simulink model "net_model_5_nodes_distributed_controllers"  (R2024b)
settings: Solver=FixedStepAuto  StartTime=0.0  StopTime=n_max  FixedStep=1  RelTol=1e-3
values from neighbouring files (symbols this model uses):
  A_ctrl = zeros(n, n, n_of_systems)    [compute_controller.m]    (also in distributed_sw_stable_ctrl_sparse_slow.mat = [-2.40828892384e-08 -0.401671155219 -3.56889576468e-19 -4.25)
  B_ctrl = -L    [compute_controller.m]    (also in distributed_sw_stable_ctrl_sparse_slow.mat = [1.00000002408 3.28131707351e-09 3.56889576468e-19 -1.412131)
  C_ctrl = J    [compute_controller.m]    (also in distributed_sw_stable_ctrl_sparse_slow.mat = [-0.301574287938 -5.67211227989e-16 -0.0985259199916 4.99277)
  D_ctrl = zeros(m, p, n_of_systems)    [compute_controller.m]    (also in distributed_sw_stable_ctrl_sparse_slow.mat = [0 0 0 0 0 0 0 0 0 0 0 0 ... (450 elements, 5x10x9)])
  n_T_local = 5    [main.m]
  node_1_0 = pi / 180 * [5, 0]'    [main.m]
  node_2_0 = pi / 180 * [-8, 0]'    [main.m]
  node_3_0 = pi / 180 * [2, 0]'    [main.m]
  node_4_0 = pi / 180 * [-8, 0]'    [main.m]
  node_5_0 = pi / 180 * [-3, 0]'    [main.m]
  T_A = zeros(n_states, n_states, n_of_systems)    [compute_controller.m]    (also in distributed_sw_stable_ctrl_sparse_slow.mat = [0 0 0 0 0 0 0 0 0 0 0 0 ... (225 elements, 5x5x9)])
  T_B = zeros(n_states, 10, n_of_systems)    [compute_controller.m]    (also in distributed_sw_stable_ctrl_sparse_slow.mat = [0 0 0 0 0 0 0 0 0 0 0 0 ... (450 elements, 5x10x9)])
  T_C = zeros(5, n_states, n_of_systems)    [compute_controller.m]    (also in distributed_sw_stable_ctrl_sparse_slow.mat = [0 0 0 0 0 0 0 0 0 0 0 0 ... (225 elements, 5x5x9)])
  T_D = zeros(5, 10, n_of_systems)    [compute_controller.m]    (also in distributed_sw_stable_ctrl_sparse_slow.mat = [0 0 0 0 0 0 0 0 0 0 0 0 ... (450 elements, 5x10x9)]; main.m)
undefined symbols (not defined in the file or in its folder): a, A_matrices, B, C
(part 2 of 2)

== matlab function net_model_5_nodes_distributed_controllers/Node 1/Interface ==
  data: delta_2 input; delta_3 input; delta_5 input; neigh_values output; l_1q input
function neigh_values = fcn(delta_2, delta_3, delta_5, l_1q)

    neigh_values = l_1q(2) * delta_2 + l_1q(3) * delta_3 + l_1q(5) * delta_5;

end

== matlab function net_model_5_nodes_distributed_controllers/Node 1/Node dynamics ==
  data: x_prev input; u input; x output; w input; neigh_values input; l_iq input; current_node input
function x = fcn(x_prev, u, w, neigh_values, l_iq, current_node)
    
    % current_node = 1;

%%

    hi = [0.3244
        1.5886;
        0.6224;
        1.0571;
        0.3313];

    di = [0.5650;
        0.7844;
        0.7347;
        0.5060;
        0.6686];

    dt = 0.2;
%%

    a21 = -hi(current_node) * dt * sum(l_iq);
    a22 = 1 - hi(current_node) * di(current_node) * dt;

    A = [1, dt;
        a21, a22];

    x = A * x_prev + [0 1]' * (u + w + hi(current_node) * dt * neigh_values);
    
end

== matlab function net_model_5_nodes_distributed_controllers/Node 3/Interface ==
  data: delta_1 input; neigh_values output; delta_4 input; delta_5 input; l_3q input
function neigh_values = fcn(delta_1, delta_4, delta_5, l_3q)

    neigh_values = l_3q(1) * delta_1 + l_3q(4) * delta_4 + l_3q(5) * delta_5;

end

== matlab function net_model_5_nodes_distributed_controllers/Node 3/Node dynamics ==
  data: x_prev input; u input; x output; w input; neigh_values input; l_iq input; current_node input
function x = fcn(x_prev, u, w, neigh_values, l_iq, current_node)
    
    % current_node = 1;

%%

    hi = [0.3244
        1.5886;
        0.6224;
        1.0571;
        0.3313];

    di = [0.5650;
        0.7844;
        0.7347;
        0.5060;
        0.6686];
    dt = 0.2;
%%

    a21 = -hi(current_node) * dt * sum(l_iq);
    a22 = 1 - hi(current_node) * di(current_node) * dt;

    A = [1, dt;
        a21, a22];

    x = A * x_prev + [0 1]' * (u + w + hi(current_node) * dt * neigh_values);
    
end

== matlab function net_model_5_nodes_distributed_controllers/Node 2/Interface ==
  data: delta_1 input; neigh_values output; delta_4 input; delta_5 input; l_2q input
function neigh_values = fcn(delta_1, delta_4, delta_5, l_2q)

    neigh_values = l_2q(1) * delta_1 + l_2q(4) * delta_4 + l_2q(5) * delta_5;

end

== matlab function net_model_5_nodes_distributed_controllers/Node 2/Node dynamics ==
  data: x_prev input; u input; x output; w input; neigh_values input; l_iq input; current_node input
function x = fcn(x_prev, u, w, neigh_values, l_iq, current_node)
    
    % current_node = 1;

%%

    hi = [0.3244
        1.5886;
        0.6224;
        1.0571;
        0.3313];

    di = [0.5650;
        0.7844;
        0.7347;
        0.5060;
        0.6686];

    dt = 0.2;
%%

    a21 = -hi(current_node) * dt * sum(l_iq);
    a22 = 1 - hi(current_node) * di(current_node) * dt;

    A = [1, dt;
        a21, a22];

    x = A * x_prev + [0 1]' * (u + w + hi(current_node) * dt * neigh_values);
    
end

== matlab function net_model_5_nodes_distributed_controllers/Node 4/Interface ==
  data: delta_2 input; neigh_values output; delta_3 input; delta_5 input; l_4q input
function neigh_values = fcn(delta_2, delta_3, delta_5, l_4q)

    neigh_values = l_4q(2) * delta_2 + l_4q(3) * delta_3 + l_4q(5) * delta_5;

end

== matlab function net_model_5_nodes_distributed_controllers/Node 4/Node dynamics ==
  data: x_prev input; u input; x output; w input; neigh_values input; l_iq input; current_node input
function x = fcn(x_prev, u, w, neigh_values, l_iq, current_node)
    
    % current_node = 1;

%%

    hi = [0.3244
        1.5886;
        0.6224;
        1.0571;
        0.3313];

    di = [0.5650;
        0.7844;
        0.7347;
        0.5060;
        0.6686];

    dt = 0.2;
%%

    a21 = -hi(current_node) * dt * sum(l_iq);
    a22 = 1 - hi(current_node) * di(current_node) * dt;

    A = [1, dt;
        a21, a22];

    x = A * x_prev + [0 1]' * (u + w + hi(current_node) * dt * neigh_values);
    
end
